simulink model "OFDM_Project_awgn_v2"  (R2025b)
settings: Solver=FixedStepDiscrete  StartTime=0.0  StopTime=100.0  RelTol=1e-3
libraries: commofdm x2, commdigbbndpm3 x2, commchan3 x1, commsink2 x1, commrandsrc3 x1
settings Model: Creator=tando  LastModifiedBy=tando

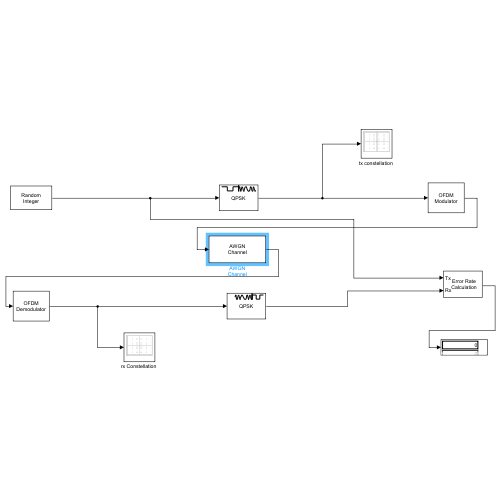
[thumbnail: Simulink's stored preview of the top-level diagram]
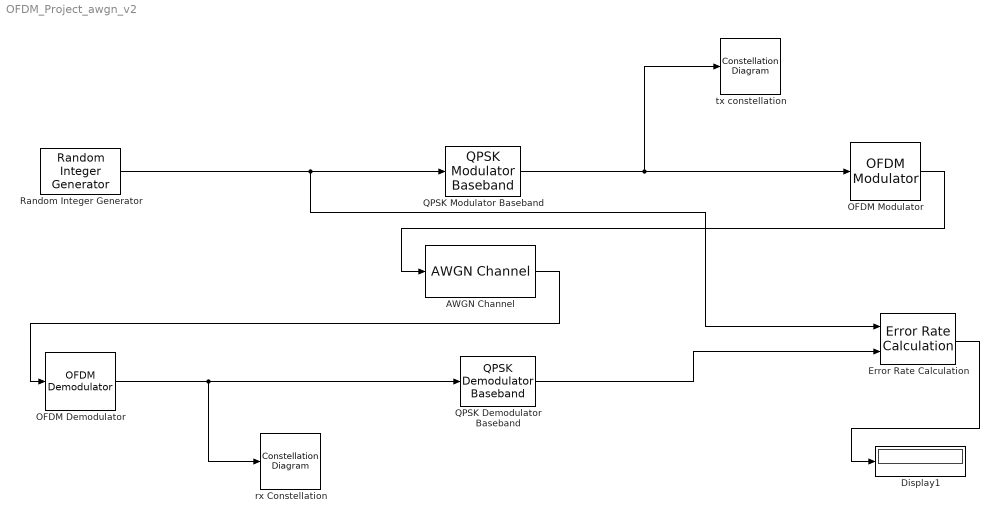
== system OFDM_Project_awgn_v2 ==
  AWGN Channel : commchan3/AWGN Channel  LegacyMode=off  NoiseMethod="Signal to noise ratio  (SNR)"  noiseMode="Signal to noise ratio  (SNR)"  EbNo=10  EsNo=10  SNR=30  BitsPerSymbol=1  SignalPower=1  SpecifySymbolPeriod=off  SamplesPerSymbol=1  SymbolPeriod=1  VarianceSource=Parameter  Variance=1  RandomStream=Global stream  Seed=67  SimulateUsing=Interpreted execution
  Display1 : Display
  Error Rate Calculation : commsink2/Error Rate Calculation  N=0  st_delay=0  cp_mode=Entire frame  subframe=[]  PMode=Port  WsName=ErrorVec  RsMode2=off  stop=off  numErr=100  maxBits=1e6
  OFDM Demodulator : commofdm/OFDM Demodulator  StatePerturbationForJacobian=1.0e-05  FFTLength=64  NumGuardBandCarriers=[6; 5]  RemoveDCCarrier=off  PilotOutputPort=off  PilotCarrierIndices=[12; 26; 40; 54]  CyclicPrefixLength=16  OversamplingFactor=1  NumSymbols=1  NumReceiveAntennas=1  SimulateUsing=Interpreted execution
  OFDM Modulator : commofdm/OFDM Modulator  StatePerturbationForJacobian=1.0e-05  FFTLength=64  NumGuardBandCarriers=[6; 5]  InsertDCNull=off  PilotInputPort=off  PilotCarrierIndices=[12; 26; 40; 54]  CyclicPrefixLength=16  Windowing=off  WindowLength=1  OversamplingFactor=1  NumSymbols=1  NumTransmitAntennas=1  SimulateUsing=Interpreted execution
  QPSK Demodulator Baseband : commdigbbndpm3/QPSK Demodulator Baseband  OutType=Integer  DecType=Hard decision  VarSource=Dialog  Variance=1  Dec=Gray  Ph=pi/4  outDtype1=Inherit via internal rule  outDtype2=Inherit via internal rule  derotateFactorWordLen=16  derotateFactorDataTypeStr=Inherit: Same word length as input  derotateFactorLastDataTypeStr=Inherit: Same word length as input
  QPSK Modulator Baseband : commdigbbndpm3/QPSK Modulator Baseband  InType=Integer  Enc=Gray  Ph=pi/4  outDtype=double  outWordLen=16  outUDDataType=sfix(16)  outFracLenMode=Best precision  outFracLen=15  outDataTypeStr=double  outLastDataTypeStr=double
  Random Integer Generator : commrandsrc3/Random Integer Generator  SetSize=4  SeedSource=Auto  Seed=0  SampleTime=1  SamplesPerFrame=53  OutputDataType=double  SimulateUsing=Interpreted execution
  "rx Constellation " : ConstellationDiagram  WindowPosition=[468.000000,180.000000,600.000000,600.000000,]  ScopeFrameLocation=window
  "tx constellation " : ConstellationDiagram  WindowPosition=[468.000000,180.000000,600.000000,600.000000,]  ScopeFrameLocation=window
  wires:
  Random Integer Generator/1 -> Error Rate Calculation/1, QPSK Modulator Baseband/1
  QPSK Modulator Baseband/1 -> OFDM Modulator/1, "tx constellation "/1
  OFDM Modulator/1 -> AWGN Channel/1
  AWGN Channel/1 -> OFDM Demodulator/1
  OFDM Demodulator/1 -> "rx Constellation "/1, QPSK Demodulator Baseband/1
  QPSK Demodulator Baseband/1 -> Error Rate Calculation/2
  Error Rate Calculation/1 -> Display1/1
